simulink model "HANcoder_E407_TTA_Controller_v3"  (R2018b)
settings: Solver=FixedStepDiscrete  StartTime=0.0  StopTime=1  FixedStep=0.01  RelTol=1e-3
PreLoadFcn:
  | librarySetup
  | eval([bdroot,'_startup']) %Calling [modelName]_startup.m
values from neighbouring files (symbols this model uses):
  basic_cycle_duration_bc0 = TM_Reset_Board   + COMP_duration    (= 212)    [HANcoder_E407_TTA_Controller_v3_startup.m]
  basic_cycle_duration_bc1 = TM_Reset_Var_bc1 + COMP_duration    (= 288)    [HANcoder_E407_TTA_Controller_v3_startup.m]
  comm_delay_estimation1 = round(comm_delay_measured1*hardware_granularity/frequency_IRQ)    [HANcoder_E407_TTA_Controller_v3_startup.m]
  comm_delay_estimation2 = round(comm_delay_measured2*hardware_granularity/frequency_IRQ)    [HANcoder_E407_TTA_Controller_v3_startup.m]
  COMM_Period = 40    [HANcoder_E407_TTA_Controller_v3_startup.m]
  COMM_Phase1 = 5    [HANcoder_E407_TTA_Controller_v3_startup.m]
  COMM_Phase2 = 8    [HANcoder_E407_TTA_Controller_v3_startup.m]
  COMP_duration = 4    [HANcoder_E407_TTA_Controller_v3_startup.m]
  Controller1_Board = 1    [HANcoder_E407_TTA_Controller_v3_startup.m]
  Controller2_Board = 2    [HANcoder_E407_TTA_Controller_v3_startup.m]
  Controller3_Board = 3    [HANcoder_E407_TTA_Controller_v3_startup.m]
  delta_a_set = Simulink.Parameter    [HANcoder_E407_TTA_Controller_v3_startup.m]
  delta_f_set = Simulink.Parameter    [HANcoder_E407_TTA_Controller_v3_startup.m]
  delta_max = 1    [HANcoder_E407_TTA_Controller_v3_startup.m]
  delta_min = -1    [HANcoder_E407_TTA_Controller_v3_startup.m]
  delta_precision = 6    [HANcoder_E407_TTA_Controller_v3_startup.m]
  e_width = 0.1    [HANcoder_E407_TTA_Controller_v3_startup.m]
  frequency_IRQ = 100    [HANcoder_E407_TTA_Controller_v3_startup.m]
  HANtuneOverride = Simulink.Parameter    [HANcoder_E407_TTA_Controller_v3_startup.m]
  hardware_granularity = 1000000    [HANcoder_E407_TTA_Controller_v3_startup.m]
  I_a = 2.25    [HANcoder_E407_TTA_Controller_v3_startup.m]
  I_f = 2.25    [HANcoder_E407_TTA_Controller_v3_startup.m]
  idle_time_init = basic_cycle_duration_bc0 + basic_cycle_duration_bc1    (= 500)    [HANcoder_E407_TTA_Controller_v3_startup.m]
  Input_Gen_Board = 4    [HANcoder_E407_TTA_Controller_v3_startup.m]
  LA_Clock_Gr = 1    [HANcoder_E407_TTA_Controller_v3_startup.m]
  LA_COMM_Err = 0    [HANcoder_E407_TTA_Controller_v3_startup.m]
  LA_MEX_Flag = 0    [HANcoder_E407_TTA_Controller_v3_startup.m]
  LA_Task_Act = 1    [HANcoder_E407_TTA_Controller_v3_startup.m]
  m_v = 100.0    (= 100)    [HANcoder_E407_TTA_Controller_v3_startup.m]
  Master_Role = 1    [HANcoder_E407_TTA_Controller_v3_startup.m]
  matrix_cycle_duration = basic_cycle_duration_bc0 + basic_cycle_duration_bc1    (= 500)    [HANcoder_E407_TTA_Controller_v3_startup.m]
  matrix_rows = 2    [HANcoder_E407_TTA_Controller_v3_startup.m]
  max_num_msgs_CAN1 = 2^Tx_bit_number-1    (= 7)    [HANcoder_E407_TTA_Controller_v3_startup.m]
  max_num_msgs_CAN2 = max_num_msgs_CAN1    (= 7)    [HANcoder_E407_TTA_Controller_v3_startup.m]
  OutControl1_ID = 23    [HANcoder_E407_TTA_Controller_v3_startup.m]
  OutControl2_ID = 24    [HANcoder_E407_TTA_Controller_v3_startup.m]
  OutEmulator_ID = 25    [HANcoder_E407_TTA_Controller_v3_startup.m]
  R_al = 0.10    (= 0.1)    [HANcoder_E407_TTA_Controller_v3_startup.m]
  R_ar = 0.10    (= 0.1)    [HANcoder_E407_TTA_Controller_v3_startup.m]
  R_fl = 0.10    (= 0.1)    [HANcoder_E407_TTA_Controller_v3_startup.m]
  R_fr = 0.10    (= 0.1)    [HANcoder_E407_TTA_Controller_v3_startup.m]
  SensorValues_ID = 22    [HANcoder_E407_TTA_Controller_v3_startup.m]
  SetValues_ID = 21    [HANcoder_E407_TTA_Controller_v3_startup.m]
  Slave_Role = 2    [HANcoder_E407_TTA_Controller_v3_startup.m]
  speed_k_d = Simulink.Parameter    [HANcoder_E407_TTA_Controller_v3_startup.m]
  speed_k_i = Simulink.Parameter    [HANcoder_E407_TTA_Controller_v3_startup.m]
  speed_k_p = Simulink.Parameter    [HANcoder_E407_TTA_Controller_v3_startup.m]
  speed_max = 10    [HANcoder_E407_TTA_Controller_v3_startup.m]
  speed_min = -10    [HANcoder_E407_TTA_Controller_v3_startup.m]
  speed_precision = 3    [HANcoder_E407_TTA_Controller_v3_startup.m]
  Sync_ID = 1    [HANcoder_E407_TTA_Controller_v3_startup.m]
  tau_max = 5    [HANcoder_E407_TTA_Controller_v3_startup.m]
  tau_min = -5    [HANcoder_E407_TTA_Controller_v3_startup.m]
  tau_range = abs(tau_max) + abs(tau_min)    [HANcoder_E407_TTA_Controller_v3_startup.m]
  theta_max = 2    [HANcoder_E407_TTA_Controller_v3_startup.m]
  theta_min = -2    [HANcoder_E407_TTA_Controller_v3_startup.m]
  theta_precision = 5    [HANcoder_E407_TTA_Controller_v3_startup.m]
  Tl_a = 0.6    [HANcoder_E407_TTA_Controller_v3_startup.m]
  Tl_f = 0.6    [HANcoder_E407_TTA_Controller_v3_startup.m]
  TM_Check_Output_Control1 = TM_COMM_Output_Control1 + COMM_duration    (= 188)    [HANcoder_E407_TTA_Controller_v3_startup.m]
  TM_Check_Output_Control2 = TM_COMM_Output_Control2 + COMM_duration    (= 232)    [HANcoder_E407_TTA_Controller_v3_startup.m]
  TM_Check_Output_Emulator = TM_COMM_Output_Emulator + COMM_duration    (= 280)    [HANcoder_E407_TTA_Controller_v3_startup.m]
  TM_Check_Sensor_Values = TM_COMM_Sensor_Values + COMM_duration    (= 132)    [HANcoder_E407_TTA_Controller_v3_startup.m]
  TM_Check_Set_Values = TM_COMM_Set_Values + COMM_duration    (= 88)    [HANcoder_E407_TTA_Controller_v3_startup.m]
  TM_Check_Sync = TM_COMM_Sync   + COMM_duration    (= 40)    [HANcoder_E407_TTA_Controller_v3_startup.m]
  TM_Check_TOuts = TM_Count_Vote3 + COMP_duration    (= 196)    [HANcoder_E407_TTA_Controller_v3_startup.m]
  TM_Check_Vote1 = TM_COMM_Vote1  + COMM_duration    (= 92)    [HANcoder_E407_TTA_Controller_v3_startup.m]
  TM_Check_Vote2 = TM_COMM_Vote2  + COMM_duration    (= 140)    [HANcoder_E407_TTA_Controller_v3_startup.m]
  TM_Check_Vote3 = TM_COMM_Vote3  + COMM_duration    (= 188)    [HANcoder_E407_TTA_Controller_v3_startup.m]
  TM_COMM_Output_Control1 = TM_Velocity + COMP_duration    (= 148)    [HANcoder_E407_TTA_Controller_v3_startup.m]
  TM_COMM_Output_Control2 = TM_Check_Output_Control1 + COMP_duration    (= 192)    [HANcoder_E407_TTA_Controller_v3_startup.m]
  TM_COMM_Output_Emulator = TM_TMR + COMP_duration    (= 240)    [HANcoder_E407_TTA_Controller_v3_startup.m]
  TM_COMM_Sensor_Values = TM_Check_Set_Values + COMP_duration    (= 92)    [HANcoder_E407_TTA_Controller_v3_startup.m]
  TM_COMM_Set_Values = TM_Update_LT + COMP_duration    (= 48)    [HANcoder_E407_TTA_Controller_v3_startup.m]
  TM_COMM_Sync = basic_cycle_start    (= 0)    [HANcoder_E407_TTA_Controller_v3_startup.m]
  TM_COMM_Vote1 = TM_Vote_Dec    + COMP_duration    (= 52)    [HANcoder_E407_TTA_Controller_v3_startup.m]
  TM_COMM_Vote2 = TM_Count_Vote1 + COMP_duration    (= 100)    [HANcoder_E407_TTA_Controller_v3_startup.m]
  TM_COMM_Vote3 = TM_Count_Vote2 + COMP_duration    (= 148)    [HANcoder_E407_TTA_Controller_v3_startup.m]
  TM_Count_Vote1 = TM_Check_Vote1 + COMP_duration    (= 96)    [HANcoder_E407_TTA_Controller_v3_startup.m]
  TM_Count_Vote2 = TM_Check_Vote2 + COMP_duration    (= 144)    [HANcoder_E407_TTA_Controller_v3_startup.m]
  TM_Count_Vote3 = TM_Check_Vote3 + COMP_duration    (= 192)    [HANcoder_E407_TTA_Controller_v3_startup.m]
  TM_Data_bc0 = TM_COMM_Sync    (= 0)    [HANcoder_E407_TTA_Controller_v3_startup.m]
  TM_Data_bc1 = TM_Data_bc0(1:3)    [HANcoder_E407_TTA_Controller_v3_startup.m]
  TM_New_Master = TM_Check_TOuts + COMP_duration    (= 200)    [HANcoder_E407_TTA_Controller_v3_startup.m]
  TM_Reset_Board = TM_Reset_Var   + COMP_duration    (= 208)    [HANcoder_E407_TTA_Controller_v3_startup.m]
  TM_Reset_Var = TM_New_Master  + COMP_duration    (= 204)    [HANcoder_E407_TTA_Controller_v3_startup.m]
  TM_Reset_Var_bc1 = TM_Check_Output_Emulator + COMP_duration    (= 284)    [HANcoder_E407_TTA_Controller_v3_startup.m]
  TM_Steer = TM_Check_Sensor_Values + COMP_duration    (= 136)    [HANcoder_E407_TTA_Controller_v3_startup.m]
  TM_TMR = TM_Check_Output_Control2 + COMP_duration    (= 236)    [HANcoder_E407_TTA_Controller_v3_startup.m]
  TM_Torque = TM_Steer + COMP_duration    (= 140)    [HANcoder_E407_TTA_Controller_v3_startup.m]
  TM_Type_bc0 = COMM    (= 0)    [HANcoder_E407_TTA_Controller_v3_startup.m]
  TM_Type_bc1 = TM_Type_bc0(1:3)    [HANcoder_E407_TTA_Controller_v3_startup.m]
  TM_Update_LT = TM_Check_Sync  + COMP_duration    (= 44)    [HANcoder_E407_TTA_Controller_v3_startup.m]
  TM_Velocity = TM_Torque + COMP_duration    (= 144)    [HANcoder_E407_TTA_Controller_v3_startup.m]
  TM_Vote_Dec = TM_Update_LT   + COMP_duration    (= 48)    [HANcoder_E407_TTA_Controller_v3_startup.m]
  torque_a_k_d = Simulink.Parameter    [HANcoder_E407_TTA_Controller_v3_startup.m]
  torque_a_k_i = Simulink.Parameter    [HANcoder_E407_TTA_Controller_v3_startup.m]
  torque_a_k_p = Simulink.Parameter    [HANcoder_E407_TTA_Controller_v3_startup.m]
  torque_f_k_d = Simulink.Parameter    [HANcoder_E407_TTA_Controller_v3_startup.m]
  torque_f_k_i = Simulink.Parameter    [HANcoder_E407_TTA_Controller_v3_startup.m]
  torque_f_k_p = Simulink.Parameter    [HANcoder_E407_TTA_Controller_v3_startup.m]
  torque_precision = 4    [HANcoder_E407_TTA_Controller_v3_startup.m]
  v_set = Simulink.Parameter    [HANcoder_E407_TTA_Controller_v3_startup.m]
  Vehicle_Em_Board = 5    [HANcoder_E407_TTA_Controller_v3_startup.m]
  Vote1_ID = 11    [HANcoder_E407_TTA_Controller_v3_startup.m]
  Vote2_ID = 12    [HANcoder_E407_TTA_Controller_v3_startup.m]
  Vote3_ID = 13    [HANcoder_E407_TTA_Controller_v3_startup.m]
undefined symbols (not defined in the file or in its folder): A0, A1, A2, A3, A4, CON2
libraries: hdlsllib x352, HANcoder_STM32_Target x25, simulink x3, simulink_extras x1
(part 18 of 32)

== system HANcoder_E407_TTA_Controller_v3/HANcoder STM32 Target - E407-STM32 algorithm/Global Ticks Increment/CAN Management/Matrix Cycle Manager/Controller Matrix Cycle/controller basic cycle 0/COMP Task - Vote3 check/Process_Messages/Demux message CAN1 and check coherence1 ==
  CAN2_Rx_msg : Inport  OutDataTypeStr=Bus: msg_buffer_type
  expected_board_id : Inport  Port=2
  Enable : EnablePort
  Bus Creator : BusCreator  Inputs=8  OutDataTypeStr=Bus: msg_buffer_type
  Bus Selector : BusSelector  OutputSignals=Buffer_1,Buffer_2,Buffer_3,Buffer_4,Buffer_5,Buffer_6,Buffer_7,Buffer_8
  Cast To Double : DataTypeConversion  OutDataTypeStr=double
  Constant : Constant  Value=0  OutDataTypeStr=uint8
  Equal : RelationalOperator  Operator===  OutDataTypeStr=boolean  RndMeth=Simplest
  Subsystem : Subsystem
  Terminator : Terminator
  Terminator1 : Terminator
  msg_count>2_DEBUG : Subsystem
  CAN2_msg_coherent : Outport  OutputWhenDisabled=reset  InitialOutput=0
  Msg_Count_CAN2 : Outport  Port=2
  CAN2_msg : Outport  Port=3  OutDataTypeStr=Bus: msg_buffer_type
  wires:
  Bus Selector/2 -> Bus Creator/2  "<Buffer_2>"
  Bus Selector/3 -> Bus Creator/3  "<Buffer_3>"
  CAN2_Rx_msg/1 -> Bus Selector/1
  Equal/1 -> CAN2_msg_coherent/1
  expected_board_id/1 -> Equal/2
  Bus Selector/6 -> Bus Creator/6  "<Buffer_6>"
  Bus Selector/5 -> Bus Creator/5  "<Buffer_5>"
  Bus Selector/7 -> Bus Creator/7  "<Buffer_7>"
  Bus Selector/8 -> Bus Creator/8  "<Buffer_8>"
  Bus Selector/4 -> Bus Creator/4  "<Buffer_4>"
  Subsystem/3(board_id) -> Equal/1  "Rx_id_vote3_CAN2"
  Bus Selector/1 -> Cast To Double/1, Subsystem/1(Msg_Temporal_Data)  "<Buffer_1>"
  Subsystem/2(msg_count) -> Msg_Count_CAN2/1, msg_count>2_DEBUG/1(msg_c)  "Rx_mc_vote3_CAN2"
  Bus Creator/1 -> CAN2_msg/1
  Constant/1 -> Bus Creator/1
  Subsystem/1(basic_cycle) -> Terminator/1  "Rx_bc_vote3_CAN2"
  Cast To Double/1 -> Terminator1/1  "Rx_temporal_vote3_CAN2"

== system HANcoder_E407_TTA_Controller_v3/HANcoder STM32 Target - E407-STM32 algorithm/Global Ticks Increment/CAN Management/Matrix Cycle Manager/Controller Matrix Cycle/controller basic cycle 1/COMM Task - Output Control1/Reception substasks/RX buffers update ==
  note: CAN2
  note: CAN1
  note: Reception end - Set RxID and Reset CAN buffer flags
  note: Reset Rx buffers
  note: Wait until new message
      | arrives
  note: Reception ID
      |    Sync Msg: 1
      |    Vote Node 1: 11
      |    Vote Node 2: 12
      |    Vote Node 3: 13
  note: Reset RX Buffer Flag
  note: Wait until new message
      | arrives
  note: Reception ID
      |    Sync Msg: 1
      |    Vote Node 1: 11
      |    Vote Node 2: 12
      |    Vote Node 3: 13
  note: Reset RX Buffer Flag
  Rx_ID : Inport
  Enable : EnablePort
  Cast13 : DataTypeConversion  OutDataTypeStr=uint32
  Cast14 : DataTypeConversion  OutDataTypeStr=boolean
  Cast15 : DataTypeConversion  OutDataTypeStr=uint8
  Cast3 : DataTypeConversion  OutDataTypeStr=uint32
  Cast5 : DataTypeConversion  OutDataTypeStr=boolean
  Cast6 : DataTypeConversion  OutDataTypeStr=uint8
  Data Store Write : DataStoreWrite  DataStoreName=Msg_Rx
  Data Store Write11 : DataStoreWrite  DataStoreName=RxID_CAN2
  Data Store Write12 : DataStoreWrite  DataStoreName=Rx_State_CAN2
  Data Store Write2 : DataStoreWrite  DataStoreName=New_Msg_Ready_CAN1
  Data Store Write3 : DataStoreWrite  DataStoreName=new_msg_Rx
  Data Store Write6 : DataStoreWrite  DataStoreName=RxID_CAN1
  Data Store Write7 : DataStoreWrite  DataStoreName=Rx_State_CAN1
  Data Store Write9 : DataStoreWrite  DataStoreName=New_Msg_Ready_CAN2
  RESET1 : Constant  Value=0
  RESET2 : Constant  Value=0
  RESET_CAN1_new_buffer : Constant  Value=0
  RESET_CAN2_new_buffer : Constant  Value=0
  RESET_Msg_Rx : Constant  Value=0  OutDataTypeStr=Bus: msg_buffer_type
  RESET_new_msg_Rx : Constant  Value=0  OutDataTypeStr=boolean
  wires:
  Cast3/1 -> Data Store Write6/1
  RESET1/1 -> Cast5/1
  Cast5/1 -> Data Store Write2/1
  RESET_Msg_Rx/1 -> Data Store Write/1
  RESET_new_msg_Rx/1 -> Data Store Write3/1
  RESET_CAN1_new_buffer/1 -> Cast6/1
  Cast6/1 -> Data Store Write7/1
  Cast15/1 -> Data Store Write12/1
  RESET_CAN2_new_buffer/1 -> Cast15/1
  Cast14/1 -> Data Store Write9/1
  RESET2/1 -> Cast14/1
  Rx_ID/1 -> Cast13/1, Cast3/1
  Cast13/1 -> Data Store Write11/1

== system HANcoder_E407_TTA_Controller_v3/HANcoder STM32 Target - E407-STM32 algorithm/Global Ticks Increment/CAN Management/Matrix Cycle Manager/Controller Matrix Cycle/controller basic cycle 1/COMM Task - Output Control1/Transmission subtasks/Check msg transmission CAN1 ==
  note: In the next tick, a message will be
      | sent through CAN1
  note: A message should be sent during
      | this tick through CAN1
  note: The TX buffers are updated one tick
      | before the message is sent
  Local Time : Inport
  Time Mark : Inport  Port=2
  Tx_ID : Inport  Port=3
  Value Domain Msg : Inport  Port=4
  Enable : EnablePort
  Constant11 : Constant  Value=0
  Constant22 : Constant
  Constant24 : Constant  Value=COMM_Phase1
  Constant27 : Constant  Value=COMM_Phase1
  Constant8 : Constant  Value=0
  Equal4 : RelationalOperator  Operator===  OutDataTypeStr=boolean  RndMeth=Simplest
  Equal7 : RelationalOperator  Operator===  OutDataTypeStr=boolean  RndMeth=Simplest
  Minus : Sum  Inputs=++-
  Minus1 : Sum  Inputs=+-
  Mod : Math  Operator=mod  SaturateOnIntegerOverflow=on
  Mod1 : Math  Operator=mod  SaturateOnIntegerOverflow=on
  TX buffer update CAN1 : Subsystem  Priority=20
  Send CAN1 : Outport  OutputWhenDisabled=reset  InitialOutput=0
  wires:
  Constant8/1 -> Equal4/2
  Equal7/1 -> Send CAN1/1
  Constant11/1 -> Equal7/2
  Minus1/1 -> Mod1/1
  Mod/1 -> Equal4/1
  Constant24/1 -> Mod/2
  Value Domain Msg/1 -> TX buffer update CAN1/2(Msg_Value_Data)
  Minus/1 -> Mod/1
  Constant27/1 -> Mod1/2
  Mod1/1 -> Equal7/1
  Tx_ID/1 -> TX buffer update CAN1/1(Tx_ID)
  Local Time/1 -> Minus/1, Minus1/1
  Constant22/1 -> Minus/2
  Equal4/1 -> TX buffer update CAN1/Enable
  Time Mark/1 -> Minus/3, Minus1/2

== system HANcoder_E407_TTA_Controller_v3/HANcoder STM32 Target - E407-STM32 algorithm/Global Ticks Increment/CAN Management/Matrix Cycle Manager/Controller Matrix Cycle/controller basic cycle 1/COMM Task - Output Control1/Transmission subtasks/Check msg transmission CAN2 ==
  note: The TX buffers are updated one tick
      | before the message is sent
  note: A message should be sent during
      | this tick through CAN2
  note: In the next tick, a message will be
      | sent through CAN2
  Local Time : Inport
  Time Mark : Inport  Port=2
  Tx_ID : Inport  Port=3
  Value Domain Msg : Inport  Port=4
  Enable : EnablePort
  Constant11 : Constant  Value=0
  Constant22 : Constant
  Constant24 : Constant  Value=COMM_Phase2
  Constant27 : Constant  Value=COMM_Phase2
  Constant8 : Constant  Value=0
  Equal4 : RelationalOperator  Operator===  OutDataTypeStr=boolean  RndMeth=Simplest
  Equal7 : RelationalOperator  Operator===  OutDataTypeStr=boolean  RndMeth=Simplest
  Minus : Sum  Inputs=++-
  Minus1 : Sum  Inputs=+-
  Mod : Math  Operator=mod  SaturateOnIntegerOverflow=on
  Mod1 : Math  Operator=mod  SaturateOnIntegerOverflow=on
  TX buffer update CAN2 : Subsystem  Priority=20
  Send CAN2 : Outport  OutputWhenDisabled=reset  InitialOutput=0
  wires:
  Time Mark/1 -> Minus1/2, Minus/3
  Equal4/1 -> TX buffer update CAN2/Enable
  Constant22/1 -> Minus/2
  Local Time/1 -> Minus1/1, Minus/1
  Tx_ID/1 -> TX buffer update CAN2/1(Tx_ID)
  Mod1/1 -> Equal7/1
  Constant27/1 -> Mod1/2
  Minus/1 -> Mod/1
  Value Domain Msg/1 -> TX buffer update CAN2/2(Msg_Value_Data)
  Constant24/1 -> Mod/2
  Mod/1 -> Equal4/1
  Minus1/1 -> Mod1/1
  Constant11/1 -> Equal7/2
  Equal7/1 -> Send CAN2/1
  Constant8/1 -> Equal4/2

== system HANcoder_E407_TTA_Controller_v3/HANcoder STM32 Target - E407-STM32 algorithm/Global Ticks Increment/CAN Management/Matrix Cycle Manager/Controller Matrix Cycle/controller basic cycle 1/COMM Task - Output Control1/Transmission subtasks/Msg_Value_Data_Encoded7 ==
  note: Value domain message encoding
      | <Warning!> The first buffer (from the top) is not used in transmission!
  Enable : EnablePort
  Bus Creator : BusCreator  Inputs=8  OutDataTypeStr=Bus: msg_buffer_type
  Cast : DataTypeConversion  OutDataTypeStr=uint8
  Cast1 : DataTypeConversion  OutDataTypeStr=uint8
  Constant : Constant  Value=0  OutDataTypeStr=uint8
  Constant{1,7,10,13} (4 alike) : Constant  Value=torque_precision
  Constant{5,8,11,14} (4 alike) : Constant  Value=tau_max
  Constant{6,9,12,15} (4 alike) : Constant  Value=tau_min
  Data Store Read : DataStoreRead  DataStoreName=torque_fr_set
  Data Store Read1 : DataStoreRead  DataStoreName=torque_fl_set
  Data Store Read2 : DataStoreRead  DataStoreName=torque_ar_set
  Data Store Read3 : DataStoreRead  DataStoreName=torque_al_set
  Data Store Read4 : DataStoreRead  DataStoreName=Error_SensorValues_NotRX
  Data Store Read5 : DataStoreRead  DataStoreName=Error_SetValues_NotRX
  float2uint1 : Subsystem
  float2uint2 : Subsystem
  float2uint3 : Subsystem
  float2uint4 : Subsystem
  Value_domain_msg : Outport
  wires:
  Bus Creator/1 -> Value_domain_msg/1
  Data Store Read5/1 -> Cast/1
  Data Store Read4/1 -> Cast1/1
  Cast/1 -> Bus Creator/6
  Cast1/1 -> Bus Creator/7
  Constant/1 -> Bus Creator/1, Bus Creator/8
  float2uint2/1(coded) -> Bus Creator/2
  float2uint1/1(coded) -> Bus Creator/3
  float2uint3/1(coded) -> Bus Creator/4
  float2uint4/1(coded) -> Bus Creator/5
  Data Store Read/1 -> float2uint2/2(magnitude)
  Constant1/1 -> float2uint2/1(precision)
  Constant5/1 -> float2uint2/3(magnitude_max)
  Constant6/1 -> float2uint2/4(magnitude_min)
  Constant9/1 -> float2uint1/4(magnitude_min)
  Constant8/1 -> float2uint1/3(magnitude_max)
  Constant7/1 -> float2uint1/1(precision)
  Data Store Read1/1 -> float2uint1/2(magnitude)
  Constant10/1 -> float2uint3/1(precision)
  Data Store Read2/1 -> float2uint3/2(magnitude)
  Constant11/1 -> float2uint3/3(magnitude_max)
  Constant12/1 -> float2uint3/4(magnitude_min)
  Constant13/1 -> float2uint4/1(precision)
  Data Store Read3/1 -> float2uint4/2(magnitude)
  Constant14/1 -> float2uint4/3(magnitude_max)
  Constant15/1 -> float2uint4/4(magnitude_min)

== system HANcoder_E407_TTA_Controller_v3/HANcoder STM32 Target - E407-STM32 algorithm/Global Ticks Increment/CAN Management/Matrix Cycle Manager/Controller Matrix Cycle/controller basic cycle 1/COMM Task - Output Control2/Reception substasks/RX buffers update ==
  note: Reset RX Buffer Flag
  note: Reception ID
      |    Sync Msg: 1
      |    Vote Node 1: 11
      |    Vote Node 2: 12
      |    Vote Node 3: 13
  note: Wait until new message
      | arrives
  note: Reset RX Buffer Flag
  note: Reception ID
      |    Sync Msg: 1
      |    Vote Node 1: 11
      |    Vote Node 2: 12
      |    Vote Node 3: 13
  note: Wait until new message
      | arrives
  note: Reset Rx buffers
  note: Reception end - Set RxID and Reset CAN buffer flags
  note: CAN1
  note: CAN2
  Rx_ID : Inport
  Enable : EnablePort
  Cast13 : DataTypeConversion  OutDataTypeStr=uint32
  Cast14 : DataTypeConversion  OutDataTypeStr=boolean
  Cast15 : DataTypeConversion  OutDataTypeStr=uint8
  Cast3 : DataTypeConversion  OutDataTypeStr=uint32
  Cast5 : DataTypeConversion  OutDataTypeStr=boolean
  Cast6 : DataTypeConversion  OutDataTypeStr=uint8
  Data Store Write : DataStoreWrite  DataStoreName=Msg_Rx
  Data Store Write11 : DataStoreWrite  DataStoreName=RxID_CAN2
  Data Store Write12 : DataStoreWrite  DataStoreName=Rx_State_CAN2
  Data Store Write2 : DataStoreWrite  DataStoreName=New_Msg_Ready_CAN1
  Data Store Write3 : DataStoreWrite  DataStoreName=new_msg_Rx
  Data Store Write6 : DataStoreWrite  DataStoreName=RxID_CAN1
  Data Store Write7 : DataStoreWrite  DataStoreName=Rx_State_CAN1
  Data Store Write9 : DataStoreWrite  DataStoreName=New_Msg_Ready_CAN2
  RESET1 : Constant  Value=0
  RESET2 : Constant  Value=0
  RESET_CAN1_new_buffer : Constant  Value=0
  RESET_CAN2_new_buffer : Constant  Value=0
  RESET_Msg_Rx : Constant  Value=0  OutDataTypeStr=Bus: msg_buffer_type
  RESET_new_msg_Rx : Constant  Value=0  OutDataTypeStr=boolean
  wires:
  Cast13/1 -> Data Store Write11/1
  Rx_ID/1 -> Cast3/1, Cast13/1
  RESET2/1 -> Cast14/1
  Cast14/1 -> Data Store Write9/1
  RESET_CAN2_new_buffer/1 -> Cast15/1
  Cast15/1 -> Data Store Write12/1
  Cast6/1 -> Data Store Write7/1
  RESET_CAN1_new_buffer/1 -> Cast6/1
  RESET_new_msg_Rx/1 -> Data Store Write3/1
  RESET_Msg_Rx/1 -> Data Store Write/1
  Cast5/1 -> Data Store Write2/1
  RESET1/1 -> Cast5/1
  Cast3/1 -> Data Store Write6/1

== system HANcoder_E407_TTA_Controller_v3/HANcoder STM32 Target - E407-STM32 algorithm/Global Ticks Increment/CAN Management/Matrix Cycle Manager/Controller Matrix Cycle/controller basic cycle 1/COMM Task - Output Control2/Transmission subtasks/Check msg transmission CAN1 ==
  note: The TX buffers are updated one tick
      | before the message is sent
  note: A message should be sent during
      | this tick through CAN1
  note: In the next tick, a message will be
      | sent through CAN1
  Local Time : Inport
  Time Mark : Inport  Port=2
  Tx_ID : Inport  Port=3
  Value Domain Msg : Inport  Port=4
  Enable : EnablePort
  Constant11 : Constant  Value=0
  Constant22 : Constant
  Constant24 : Constant  Value=COMM_Phase1
  Constant27 : Constant  Value=COMM_Phase1
  Constant8 : Constant  Value=0
  Equal4 : RelationalOperator  Operator===  OutDataTypeStr=boolean  RndMeth=Simplest
  Equal7 : RelationalOperator  Operator===  OutDataTypeStr=boolean  RndMeth=Simplest
  Minus : Sum  Inputs=++-
  Minus1 : Sum  Inputs=+-
  Mod : Math  Operator=mod  SaturateOnIntegerOverflow=on
  Mod1 : Math  Operator=mod  SaturateOnIntegerOverflow=on
  TX buffer update CAN1 : Subsystem  Priority=20
  Send CAN1 : Outport  OutputWhenDisabled=reset  InitialOutput=0
  wires:
  Time Mark/1 -> Minus1/2, Minus/3
  Equal4/1 -> TX buffer update CAN1/Enable
  Constant22/1 -> Minus/2
  Local Time/1 -> Minus1/1, Minus/1
  Tx_ID/1 -> TX buffer update CAN1/1(Tx_ID)
  Mod1/1 -> Equal7/1
  Constant27/1 -> Mod1/2
  Minus/1 -> Mod/1
  Value Domain Msg/1 -> TX buffer update CAN1/2(Msg_Value_Data)
  Constant24/1 -> Mod/2
  Mod/1 -> Equal4/1
  Minus1/1 -> Mod1/1
  Constant11/1 -> Equal7/2
  Equal7/1 -> Send CAN1/1
  Constant8/1 -> Equal4/2

== system HANcoder_E407_TTA_Controller_v3/HANcoder STM32 Target - E407-STM32 algorithm/Global Ticks Increment/CAN Management/Matrix Cycle Manager/Controller Matrix Cycle/controller basic cycle 1/COMM Task - Output Control2/Transmission subtasks/Check msg transmission CAN2 ==
  note: In the next tick, a message will be
      | sent through CAN2
  note: A message should be sent during
      | this tick through CAN2
  note: The TX buffers are updated one tick
      | before the message is sent
  Local Time : Inport
  Time Mark : Inport  Port=2
  Tx_ID : Inport  Port=3
  Value Domain Msg : Inport  Port=4
  Enable : EnablePort
  Constant11 : Constant  Value=0
  Constant22 : Constant
  Constant24 : Constant  Value=COMM_Phase2
  Constant27 : Constant  Value=COMM_Phase2
  Constant8 : Constant  Value=0
  Equal4 : RelationalOperator  Operator===  OutDataTypeStr=boolean  RndMeth=Simplest
  Equal7 : RelationalOperator  Operator===  OutDataTypeStr=boolean  RndMeth=Simplest
  Minus : Sum  Inputs=++-
  Minus1 : Sum  Inputs=+-
  Mod : Math  Operator=mod  SaturateOnIntegerOverflow=on
  Mod1 : Math  Operator=mod  SaturateOnIntegerOverflow=on
  TX buffer update CAN2 : Subsystem  Priority=20
  Send CAN2 : Outport  OutputWhenDisabled=reset  InitialOutput=0
  wires:
  Constant8/1 -> Equal4/2
  Equal7/1 -> Send CAN2/1
  Constant11/1 -> Equal7/2
  Minus1/1 -> Mod1/1
  Mod/1 -> Equal4/1
  Constant24/1 -> Mod/2
  Value Domain Msg/1 -> TX buffer update CAN2/2(Msg_Value_Data)
  Minus/1 -> Mod/1
  Constant27/1 -> Mod1/2
  Mod1/1 -> Equal7/1
  Tx_ID/1 -> TX buffer update CAN2/1(Tx_ID)
  Local Time/1 -> Minus/1, Minus1/1
  Constant22/1 -> Minus/2
  Equal4/1 -> TX buffer update CAN2/Enable
  Time Mark/1 -> Minus/3, Minus1/2

== system HANcoder_E407_TTA_Controller_v3/HANcoder STM32 Target - E407-STM32 algorithm/Global Ticks Increment/CAN Management/Matrix Cycle Manager/Controller Matrix Cycle/controller basic cycle 1/COMM Task - Output Control2/Transmission subtasks/Msg_Value_Data_Encoded7 ==
  note: Value domain message encoding
      | <Warning!> The first buffer (from the top) is not used in transmission!
  Enable : EnablePort
  Bus Creator : BusCreator  Inputs=8  OutDataTypeStr=Bus: msg_buffer_type
  Cast : DataTypeConversion  OutDataTypeStr=uint8
  Cast1 : DataTypeConversion  OutDataTypeStr=uint8
  Constant : Constant  Value=0  OutDataTypeStr=uint8
  Constant{1,7,10,13} (4 alike) : Constant  Value=torque_precision
  Constant{5,8,11,14} (4 alike) : Constant  Value=tau_max
  Constant{6,9,12,15} (4 alike) : Constant  Value=tau_min
  Data Store Read : DataStoreRead  DataStoreName=torque_fr_set
  Data Store Read1 : DataStoreRead  DataStoreName=torque_fl_set
  Data Store Read2 : DataStoreRead  DataStoreName=torque_ar_set
  Data Store Read3 : DataStoreRead  DataStoreName=torque_al_set
  Data Store Read4 : DataStoreRead  DataStoreName=Error_SensorValues_NotRX
  Data Store Read5 : DataStoreRead  DataStoreName=Error_SetValues_NotRX
  float2uint1 : Subsystem
  float2uint2 : Subsystem
  float2uint3 : Subsystem
  float2uint4 : Subsystem
  Value_domain_msg : Outport
  wires:
  Constant15/1 -> float2uint4/4(magnitude_min)
  Constant14/1 -> float2uint4/3(magnitude_max)
  Data Store Read3/1 -> float2uint4/2(magnitude)
  Constant13/1 -> float2uint4/1(precision)
  Constant12/1 -> float2uint3/4(magnitude_min)
  Constant11/1 -> float2uint3/3(magnitude_max)
  Data Store Read2/1 -> float2uint3/2(magnitude)
  Constant10/1 -> float2uint3/1(precision)
  Data Store Read1/1 -> float2uint1/2(magnitude)
  Constant7/1 -> float2uint1/1(precision)
  Constant8/1 -> float2uint1/3(magnitude_max)
  Constant9/1 -> float2uint1/4(magnitude_min)
  Constant6/1 -> float2uint2/4(magnitude_min)
  Constant5/1 -> float2uint2/3(magnitude_max)
  Constant1/1 -> float2uint2/1(precision)
  Data Store Read/1 -> float2uint2/2(magnitude)
  float2uint4/1(coded) -> Bus Creator/5
  float2uint3/1(coded) -> Bus Creator/4
  float2uint1/1(coded) -> Bus Creator/3
  float2uint2/1(coded) -> Bus Creator/2
  Constant/1 -> Bus Creator/8, Bus Creator/1
  Cast1/1 -> Bus Creator/7
  Cast/1 -> Bus Creator/6
  Data Store Read4/1 -> Cast1/1
  Data Store Read5/1 -> Cast/1
  Bus Creator/1 -> Value_domain_msg/1

== system HANcoder_E407_TTA_Controller_v3/HANcoder STM32 Target - E407-STM32 algorithm/Global Ticks Increment/CAN Management/Matrix Cycle Manager/Controller Matrix Cycle/controller basic cycle 1/COMM Task - Output Emulator/Reception substasks/RX buffers update ==
  note: CAN2
  note: CAN1
  note: Reception end - Set RxID and Reset CAN buffer flags
  note: Reset Rx buffers
  note: Wait until new message
      | arrives
  note: Reception ID
      |    Sync Msg: 1
      |    Vote Node 1: 11
      |    Vote Node 2: 12
      |    Vote Node 3: 13
  note: Reset RX Buffer Flag
  note: Wait until new message
      | arrives
  note: Reception ID
      |    Sync Msg: 1
      |    Vote Node 1: 11
      |    Vote Node 2: 12
      |    Vote Node 3: 13
  note: Reset RX Buffer Flag
  Rx_ID : Inport
  Enable : EnablePort
  Cast13 : DataTypeConversion  OutDataTypeStr=uint32
  Cast14 : DataTypeConversion  OutDataTypeStr=boolean
  Cast15 : DataTypeConversion  OutDataTypeStr=uint8
  Cast3 : DataTypeConversion  OutDataTypeStr=uint32
  Cast5 : DataTypeConversion  OutDataTypeStr=boolean
  Cast6 : DataTypeConversion  OutDataTypeStr=uint8
  Data Store Write : DataStoreWrite  DataStoreName=Msg_Rx
  Data Store Write11 : DataStoreWrite  DataStoreName=RxID_CAN2
  Data Store Write12 : DataStoreWrite  DataStoreName=Rx_State_CAN2
  Data Store Write2 : DataStoreWrite  DataStoreName=New_Msg_Ready_CAN1
  Data Store Write3 : DataStoreWrite  DataStoreName=new_msg_Rx
  Data Store Write6 : DataStoreWrite  DataStoreName=RxID_CAN1
  Data Store Write7 : DataStoreWrite  DataStoreName=Rx_State_CAN1
  Data Store Write9 : DataStoreWrite  DataStoreName=New_Msg_Ready_CAN2
  RESET1 : Constant  Value=0
  RESET2 : Constant  Value=0
  RESET_CAN1_new_buffer : Constant  Value=0
  RESET_CAN2_new_buffer : Constant  Value=0
  RESET_Msg_Rx : Constant  Value=0  OutDataTypeStr=Bus: msg_buffer_type
  RESET_new_msg_Rx : Constant  Value=0  OutDataTypeStr=boolean
  wires:
  Cast3/1 -> Data Store Write6/1
  RESET1/1 -> Cast5/1
  Cast5/1 -> Data Store Write2/1
  RESET_Msg_Rx/1 -> Data Store Write/1
  RESET_new_msg_Rx/1 -> Data Store Write3/1
  RESET_CAN1_new_buffer/1 -> Cast6/1
  Cast6/1 -> Data Store Write7/1
  Cast15/1 -> Data Store Write12/1
  RESET_CAN2_new_buffer/1 -> Cast15/1
  Cast14/1 -> Data Store Write9/1
  RESET2/1 -> Cast14/1
  Rx_ID/1 -> Cast13/1, Cast3/1
  Cast13/1 -> Data Store Write11/1

== system HANcoder_E407_TTA_Controller_v3/HANcoder STM32 Target - E407-STM32 algorithm/Global Ticks Increment/CAN Management/Matrix Cycle Manager/Controller Matrix Cycle/controller basic cycle 1/COMM Task - Output Emulator/Transmission subtasks/Check msg transmission CAN1 ==
  note: In the next tick, a message will be
      | sent through CAN1
  note: A message should be sent during
      | this tick through CAN1
  note: The TX buffers are updated one tick
      | before the message is sent
  Local Time : Inport
  Time Mark : Inport  Port=2
  Tx_ID : Inport  Port=3
  Value Domain Msg : Inport  Port=4
  Enable : EnablePort
  Constant11 : Constant  Value=0
  Constant22 : Constant
  Constant24 : Constant  Value=COMM_Phase1
  Constant27 : Constant  Value=COMM_Phase1
  Constant8 : Constant  Value=0
  Equal4 : RelationalOperator  Operator===  OutDataTypeStr=boolean  RndMeth=Simplest
  Equal7 : RelationalOperator  Operator===  OutDataTypeStr=boolean  RndMeth=Simplest
  Minus : Sum  Inputs=++-
  Minus1 : Sum  Inputs=+-
  Mod : Math  Operator=mod  SaturateOnIntegerOverflow=on
  Mod1 : Math  Operator=mod  SaturateOnIntegerOverflow=on
  TX buffer update CAN1 : Subsystem  Priority=20
  Send CAN1 : Outport  OutputWhenDisabled=reset  InitialOutput=0
  wires:
  Constant8/1 -> Equal4/2
  Equal7/1 -> Send CAN1/1
  Constant11/1 -> Equal7/2
  Minus1/1 -> Mod1/1
  Mod/1 -> Equal4/1
  Constant24/1 -> Mod/2
  Value Domain Msg/1 -> TX buffer update CAN1/2(Msg_Value_Data)
  Minus/1 -> Mod/1
  Constant27/1 -> Mod1/2
  Mod1/1 -> Equal7/1
  Tx_ID/1 -> TX buffer update CAN1/1(Tx_ID)
  Local Time/1 -> Minus/1, Minus1/1
  Constant22/1 -> Minus/2
  Equal4/1 -> TX buffer update CAN1/Enable
  Time Mark/1 -> Minus/3, Minus1/2

== system HANcoder_E407_TTA_Controller_v3/HANcoder STM32 Target - E407-STM32 algorithm/Global Ticks Increment/CAN Management/Matrix Cycle Manager/Controller Matrix Cycle/controller basic cycle 1/COMM Task - Output Emulator/Transmission subtasks/Check msg transmission CAN2 ==
  note: The TX buffers are updated one tick
      | before the message is sent
  note: A message should be sent during
      | this tick through CAN2
  note: In the next tick, a message will be
      | sent through CAN2
  Local Time : Inport
  Time Mark : Inport  Port=2
  Tx_ID : Inport  Port=3
  Value Domain Msg : Inport  Port=4
  Enable : EnablePort
  Constant11 : Constant  Value=0
  Constant22 : Constant
  Constant24 : Constant  Value=COMM_Phase2
  Constant27 : Constant  Value=COMM_Phase2
  Constant8 : Constant  Value=0
  Equal4 : RelationalOperator  Operator===  OutDataTypeStr=boolean  RndMeth=Simplest
  Equal7 : RelationalOperator  Operator===  OutDataTypeStr=boolean  RndMeth=Simplest
  Minus : Sum  Inputs=++-
  Minus1 : Sum  Inputs=+-
  Mod : Math  Operator=mod  SaturateOnIntegerOverflow=on
  Mod1 : Math  Operator=mod  SaturateOnIntegerOverflow=on
  TX buffer update CAN2 : Subsystem  Priority=20
  Send CAN2 : Outport  OutputWhenDisabled=reset  InitialOutput=0
  wires:
  Time Mark/1 -> Minus1/2, Minus/3
  Equal4/1 -> TX buffer update CAN2/Enable
  Constant22/1 -> Minus/2
  Local Time/1 -> Minus1/1, Minus/1
  Tx_ID/1 -> TX buffer update CAN2/1(Tx_ID)
  Mod1/1 -> Equal7/1
  Constant27/1 -> Mod1/2
  Minus/1 -> Mod/1
  Value Domain Msg/1 -> TX buffer update CAN2/2(Msg_Value_Data)
  Constant24/1 -> Mod/2
  Mod/1 -> Equal4/1
  Minus1/1 -> Mod1/1
  Constant11/1 -> Equal7/2
  Equal7/1 -> Send CAN2/1
  Constant8/1 -> Equal4/2

== system HANcoder_E407_TTA_Controller_v3/HANcoder STM32 Target - E407-STM32 algorithm/Global Ticks Increment/CAN Management/Matrix Cycle Manager/Controller Matrix Cycle/controller basic cycle 1/COMM Task - Output Emulator/Transmission subtasks/Msg_Value_Data_Encoded ==
  note: Value domain message encoding
      | <Warning!> The first buffer (from the top) is not used in transmission!
  Enable : EnablePort
  Bus Creator : BusCreator  Inputs=8  OutDataTypeStr=Bus: msg_buffer_type
  Constant : Constant  Value=0  OutDataTypeStr=uint8
  Constant{7,10..11,14} (4 alike) : Constant  Value=tau_min
  Constant{5,8,12,15} (4 alike) : Constant  Value=torque_precision
  Constant{6,9,13,16} (4 alike) : Constant  Value=tau_max
  Data Store Read1 : DataStoreRead  DataStoreName=torque_fl_set
  Data Store Read2 : DataStoreRead  DataStoreName=torque_ar_set
  Data Store Read3 : DataStoreRead  DataStoreName=torque_al_set
  Data Store Read4 : DataStoreRead  DataStoreName=error_log_1
  Data Store Read5 : DataStoreRead  DataStoreName=error_log_2
  Data Store Read6 : DataStoreRead  DataStoreName=error_log_3
  Data Store Read7 : DataStoreRead  DataStoreName=torque_fr_set
  float2uint1 : Subsystem
  float2uint2 : Subsystem
  float2uint3 : Subsystem
  float2uint4 : Subsystem
  Value_domain_msg : Outport
  wires:
  Bus Creator/1 -> Value_domain_msg/1
  Data Store Read5/1 -> Bus Creator/7
  Data Store Read6/1 -> Bus Creator/8
  Constant/1 -> Bus Creator/1
  Data Store Read4/1 -> Bus Creator/6
  Data Store Read7/1 -> float2uint2/2(magnitude)
  Constant6/1 -> float2uint2/3(magnitude_max)
  Constant5/1 -> float2uint2/1(precision)
  Constant7/1 -> float2uint2/4(magnitude_min)
  float2uint2/1(coded) -> Bus Creator/2
  Constant10/1 -> float2uint1/4(magnitude_min)
  Constant8/1 -> float2uint1/1(precision)
  Constant9/1 -> float2uint1/3(magnitude_max)
  Data Store Read1/1 -> float2uint1/2(magnitude)
  Data Store Read2/1 -> float2uint3/2(magnitude)
  Constant13/1 -> float2uint3/3(magnitude_max)
  Constant12/1 -> float2uint3/1(precision)
  Constant11/1 -> float2uint3/4(magnitude_min)
  float2uint3/1(coded) -> Bus Creator/4
  Constant14/1 -> float2uint4/4(magnitude_min)
  Constant15/1 -> float2uint4/1(precision)
  Constant16/1 -> float2uint4/3(magnitude_max)
  Data Store Read3/1 -> float2uint4/2(magnitude)
  float2uint4/1(coded) -> Bus Creator/5
  float2uint1/1(coded) -> Bus Creator/3

== system HANcoder_E407_TTA_Controller_v3/HANcoder STM32 Target - E407-STM32 algorithm/Global Ticks Increment/CAN Management/Matrix Cycle Manager/Controller Matrix Cycle/controller basic cycle 1/COMM Task - Sensor_Values/Reception substasks/RX buffers update ==
  note: Reset RX Buffer Flag
  note: Reception ID
      |    Sync Msg: 1
      |    Vote Node 1: 11
      |    Vote Node 2: 12
      |    Vote Node 3: 13
  note: Wait until new message
      | arrives
  note: Reset RX Buffer Flag
  note: Reception ID
      |    Sync Msg: 1
      |    Vote Node 1: 11
      |    Vote Node 2: 12
      |    Vote Node 3: 13
  note: Wait until new message
      | arrives
  note: Reset Rx buffers
  note: Reception end - Set RxID and Reset CAN buffer flags
  note: CAN1
  note: CAN2
  Rx_ID : Inport
  Enable : EnablePort
  Cast13 : DataTypeConversion  OutDataTypeStr=uint32
  Cast14 : DataTypeConversion  OutDataTypeStr=boolean
  Cast15 : DataTypeConversion  OutDataTypeStr=uint8
  Cast3 : DataTypeConversion  OutDataTypeStr=uint32
  Cast5 : DataTypeConversion  OutDataTypeStr=boolean
  Cast6 : DataTypeConversion  OutDataTypeStr=uint8
  Data Store Write : DataStoreWrite  DataStoreName=Msg_Rx
  Data Store Write11 : DataStoreWrite  DataStoreName=RxID_CAN2
  Data Store Write12 : DataStoreWrite  DataStoreName=Rx_State_CAN2
  Data Store Write2 : DataStoreWrite  DataStoreName=New_Msg_Ready_CAN1
  Data Store Write3 : DataStoreWrite  DataStoreName=new_msg_Rx
  Data Store Write6 : DataStoreWrite  DataStoreName=RxID_CAN1
  Data Store Write7 : DataStoreWrite  DataStoreName=Rx_State_CAN1
  Data Store Write9 : DataStoreWrite  DataStoreName=New_Msg_Ready_CAN2
  RESET1 : Constant  Value=0
  RESET2 : Constant  Value=0
  RESET_CAN1_new_buffer : Constant  Value=0
  RESET_CAN2_new_buffer : Constant  Value=0
  RESET_Msg_Rx : Constant  Value=0  OutDataTypeStr=Bus: msg_buffer_type
  RESET_new_msg_Rx : Constant  Value=0  OutDataTypeStr=boolean
  wires:
  Cast13/1 -> Data Store Write11/1
  Rx_ID/1 -> Cast3/1, Cast13/1
  RESET2/1 -> Cast14/1
  Cast14/1 -> Data Store Write9/1
  RESET_CAN2_new_buffer/1 -> Cast15/1
  Cast15/1 -> Data Store Write12/1
  Cast6/1 -> Data Store Write7/1
  RESET_CAN1_new_buffer/1 -> Cast6/1
  RESET_new_msg_Rx/1 -> Data Store Write3/1
  RESET_Msg_Rx/1 -> Data Store Write/1
  Cast5/1 -> Data Store Write2/1
  RESET1/1 -> Cast5/1
  Cast3/1 -> Data Store Write6/1

== system HANcoder_E407_TTA_Controller_v3/HANcoder STM32 Target - E407-STM32 algorithm/Global Ticks Increment/CAN Management/Matrix Cycle Manager/Controller Matrix Cycle/controller basic cycle 1/COMM Task - Sensor_Values/Transmission subtasks/Check msg transmission CAN1 ==
  note: The TX buffers are updated one tick
      | before the message is sent
  note: A message should be sent during
      | this tick through CAN1
  note: In the next tick, a message will be
      | sent through CAN1
  Local Time : Inport
  Time Mark : Inport  Port=2
  Tx_ID : Inport  Port=3
  Value Domain Msg : Inport  Port=4
  Enable : EnablePort
  Constant11 : Constant  Value=0
  Constant22 : Constant
  Constant24 : Constant  Value=COMM_Phase1
  Constant27 : Constant  Value=COMM_Phase1
  Constant8 : Constant  Value=0
  Equal4 : RelationalOperator  Operator===  OutDataTypeStr=boolean  RndMeth=Simplest
  Equal7 : RelationalOperator  Operator===  OutDataTypeStr=boolean  RndMeth=Simplest
  Minus : Sum  Inputs=++-
  Minus1 : Sum  Inputs=+-
  Mod : Math  Operator=mod  SaturateOnIntegerOverflow=on
  Mod1 : Math  Operator=mod  SaturateOnIntegerOverflow=on
  TX buffer update CAN1 : Subsystem  Priority=20
  Send CAN1 : Outport  OutputWhenDisabled=reset  InitialOutput=0
  wires:
  Time Mark/1 -> Minus1/2, Minus/3
  Equal4/1 -> TX buffer update CAN1/Enable
  Constant22/1 -> Minus/2
  Local Time/1 -> Minus1/1, Minus/1
  Tx_ID/1 -> TX buffer update CAN1/1(Tx_ID)
  Mod1/1 -> Equal7/1
  Constant27/1 -> Mod1/2
  Minus/1 -> Mod/1
  Value Domain Msg/1 -> TX buffer update CAN1/2(Msg_Value_Data)
  Constant24/1 -> Mod/2
  Mod/1 -> Equal4/1
  Minus1/1 -> Mod1/1
  Constant11/1 -> Equal7/2
  Equal7/1 -> Send CAN1/1
  Constant8/1 -> Equal4/2

== system HANcoder_E407_TTA_Controller_v3/HANcoder STM32 Target - E407-STM32 algorithm/Global Ticks Increment/CAN Management/Matrix Cycle Manager/Controller Matrix Cycle/controller basic cycle 1/COMM Task - Sensor_Values/Transmission subtasks/Check msg transmission CAN2 ==
  note: In the next tick, a message will be
      | sent through CAN2
  note: A message should be sent during
      | this tick through CAN2
  note: The TX buffers are updated one tick
      | before the message is sent
  Local Time : Inport
  Time Mark : Inport  Port=2
  Tx_ID : Inport  Port=3
  Value Domain Msg : Inport  Port=4
  Enable : EnablePort
  Constant11 : Constant  Value=0
  Constant22 : Constant
  Constant24 : Constant  Value=COMM_Phase2
  Constant27 : Constant  Value=COMM_Phase2
  Constant8 : Constant  Value=0
  Equal4 : RelationalOperator  Operator===  OutDataTypeStr=boolean  RndMeth=Simplest
  Equal7 : RelationalOperator  Operator===  OutDataTypeStr=boolean  RndMeth=Simplest
  Minus : Sum  Inputs=++-
  Minus1 : Sum  Inputs=+-
  Mod : Math  Operator=mod  SaturateOnIntegerOverflow=on
  Mod1 : Math  Operator=mod  SaturateOnIntegerOverflow=on
  TX buffer update CAN2 : Subsystem  Priority=20
  Send CAN2 : Outport  OutputWhenDisabled=reset  InitialOutput=0
  wires:
  Constant8/1 -> Equal4/2
  Equal7/1 -> Send CAN2/1
  Constant11/1 -> Equal7/2
  Minus1/1 -> Mod1/1
  Mod/1 -> Equal4/1
  Constant24/1 -> Mod/2
  Value Domain Msg/1 -> TX buffer update CAN2/2(Msg_Value_Data)
  Minus/1 -> Mod/1
  Constant27/1 -> Mod1/2
  Mod1/1 -> Equal7/1
  Tx_ID/1 -> TX buffer update CAN2/1(Tx_ID)
  Local Time/1 -> Minus/1, Minus1/1
  Constant22/1 -> Minus/2
  Equal4/1 -> TX buffer update CAN2/Enable
  Time Mark/1 -> Minus/3, Minus1/2

== system HANcoder_E407_TTA_Controller_v3/HANcoder STM32 Target - E407-STM32 algorithm/Global Ticks Increment/CAN Management/Matrix Cycle Manager/Controller Matrix Cycle/controller basic cycle 1/COMM Task - Sensor_Values/Transmission subtasks/Msg_Value_Data_Encoded6 ==
  note: <!> This is properly defined in vehicle emulator matrix cycle
  note: Value domain message encoding
      | <Warning!> The first buffer (from the top) is not used in transmission!
  Enable : EnablePort
  Bus Creator : BusCreator  Inputs=8  OutDataTypeStr=Bus: msg_buffer_type
  Constant : Constant  Value=0  OutDataTypeStr=uint8
  Constant{1,7,10,13} (4 alike) : Constant  Value=theta_precision
  Constant{5,8,11,14} (4 alike) : Constant  Value=theta_max
  Constant{6,9,12,15} (4 alike) : Constant  Value=theta_min
  Constant{2..4,16} (4 alike) : Constant  Value=0
  float2uint1 : Subsystem
  float2uint2 : Subsystem
  float2uint3 : Subsystem
  float2uint4 : Subsystem
  Value_domain_msg : Outport
  wires:
  Bus Creator/1 -> Value_domain_msg/1
  Constant2/1 -> float2uint2/2(magnitude)
  Constant1/1 -> float2uint2/1(precision)
  Constant/1 -> Bus Creator/1, Bus Creator/6, Bus Creator/7, Bus Creator/8
  float2uint2/1(coded) -> Bus Creator/2
  Constant5/1 -> float2uint2/3(magnitude_max)
  Constant6/1 -> float2uint2/4(magnitude_min)
  Constant9/1 -> float2uint1/4(magnitude_min)
  Constant8/1 -> float2uint1/3(magnitude_max)
  Constant7/1 -> float2uint1/1(precision)
  Constant3/1 -> float2uint1/2(magnitude)
  float2uint1/1(coded) -> Bus Creator/3
  Constant4/1 -> float2uint3/2(magnitude)
  Constant10/1 -> float2uint3/1(precision)
  Constant11/1 -> float2uint3/3(magnitude_max)
  Constant12/1 -> float2uint3/4(magnitude_min)
  float2uint3/1(coded) -> Bus Creator/4
  Constant15/1 -> float2uint4/4(magnitude_min)
  Constant14/1 -> float2uint4/3(magnitude_max)
  Constant13/1 -> float2uint4/1(precision)
  Constant16/1 -> float2uint4/2(magnitude)
  float2uint4/1(coded) -> Bus Creator/5

== system HANcoder_E407_TTA_Controller_v3/HANcoder STM32 Target - E407-STM32 algorithm/Global Ticks Increment/CAN Management/Matrix Cycle Manager/Controller Matrix Cycle/controller basic cycle 1/COMM Task - Set_Values/Reception substasks/RX buffers update ==
  note: CAN2
  note: CAN1
  note: Reception end - Set RxID and Reset CAN buffer flags
  note: Reset Rx buffers
  note: Wait until new message
      | arrives
  note: Reception ID
      |    Sync Msg: 1
      |    Vote Node 1: 11
      |    Vote Node 2: 12
      |    Vote Node 3: 13
  note: Reset RX Buffer Flag
  note: Wait until new message
      | arrives
  note: Reception ID
      |    Sync Msg: 1
      |    Vote Node 1: 11
      |    Vote Node 2: 12
      |    Vote Node 3: 13
  note: Reset RX Buffer Flag
  Rx_ID : Inport
  Enable : EnablePort
  Cast13 : DataTypeConversion  OutDataTypeStr=uint32
  Cast14 : DataTypeConversion  OutDataTypeStr=boolean
  Cast15 : DataTypeConversion  OutDataTypeStr=uint8
  Cast3 : DataTypeConversion  OutDataTypeStr=uint32
  Cast5 : DataTypeConversion  OutDataTypeStr=boolean
  Cast6 : DataTypeConversion  OutDataTypeStr=uint8
  Data Store Write : DataStoreWrite  DataStoreName=Msg_Rx
  Data Store Write11 : DataStoreWrite  DataStoreName=RxID_CAN2
  Data Store Write12 : DataStoreWrite  DataStoreName=Rx_State_CAN2
  Data Store Write2 : DataStoreWrite  DataStoreName=New_Msg_Ready_CAN1
  Data Store Write3 : DataStoreWrite  DataStoreName=new_msg_Rx
  Data Store Write6 : DataStoreWrite  DataStoreName=RxID_CAN1
  Data Store Write7 : DataStoreWrite  DataStoreName=Rx_State_CAN1
  Data Store Write9 : DataStoreWrite  DataStoreName=New_Msg_Ready_CAN2
  RESET1 : Constant  Value=0
  RESET2 : Constant  Value=0
  RESET_CAN1_new_buffer : Constant  Value=0
  RESET_CAN2_new_buffer : Constant  Value=0
  RESET_Msg_Rx : Constant  Value=0  OutDataTypeStr=Bus: msg_buffer_type
  RESET_new_msg_Rx : Constant  Value=0  OutDataTypeStr=boolean
  wires:
  Cast3/1 -> Data Store Write6/1
  RESET1/1 -> Cast5/1
  Cast5/1 -> Data Store Write2/1
  RESET_Msg_Rx/1 -> Data Store Write/1
  RESET_new_msg_Rx/1 -> Data Store Write3/1
  RESET_CAN1_new_buffer/1 -> Cast6/1
  Cast6/1 -> Data Store Write7/1
  Cast15/1 -> Data Store Write12/1
  RESET_CAN2_new_buffer/1 -> Cast15/1
  Cast14/1 -> Data Store Write9/1
  RESET2/1 -> Cast14/1
  Rx_ID/1 -> Cast13/1, Cast3/1
  Cast13/1 -> Data Store Write11/1

== system HANcoder_E407_TTA_Controller_v3/HANcoder STM32 Target - E407-STM32 algorithm/Global Ticks Increment/CAN Management/Matrix Cycle Manager/Controller Matrix Cycle/controller basic cycle 1/COMM Task - Set_Values/Transmission subtasks/Check msg transmission CAN1 ==
  note: In the next tick, a message will be
      | sent through CAN1
  note: A message should be sent during
      | this tick through CAN1
  note: The TX buffers are updated one tick
      | before the message is sent
  Local Time : Inport
  Time Mark : Inport  Port=2
  Tx_ID : Inport  Port=3
  Value Domain Msg : Inport  Port=4
  Enable : EnablePort
  Constant11 : Constant  Value=0
  Constant22 : Constant
  Constant24 : Constant  Value=COMM_Phase1
  Constant27 : Constant  Value=COMM_Phase1
  Constant8 : Constant  Value=0
  Equal4 : RelationalOperator  Operator===  OutDataTypeStr=boolean  RndMeth=Simplest
  Equal7 : RelationalOperator  Operator===  OutDataTypeStr=boolean  RndMeth=Simplest
  Minus : Sum  Inputs=++-
  Minus1 : Sum  Inputs=+-
  Mod : Math  Operator=mod  SaturateOnIntegerOverflow=on
  Mod1 : Math  Operator=mod  SaturateOnIntegerOverflow=on
  TX buffer update CAN1 : Subsystem  Priority=20
  Send CAN1 : Outport  OutputWhenDisabled=reset  InitialOutput=0
  wires:
  Constant8/1 -> Equal4/2
  Equal7/1 -> Send CAN1/1
  Constant11/1 -> Equal7/2
  Minus1/1 -> Mod1/1
  Mod/1 -> Equal4/1
  Constant24/1 -> Mod/2
  Value Domain Msg/1 -> TX buffer update CAN1/2(Msg_Value_Data)
  Minus/1 -> Mod/1
  Constant27/1 -> Mod1/2
  Mod1/1 -> Equal7/1
  Tx_ID/1 -> TX buffer update CAN1/1(Tx_ID)
  Local Time/1 -> Minus/1, Minus1/1
  Constant22/1 -> Minus/2
  Equal4/1 -> TX buffer update CAN1/Enable
  Time Mark/1 -> Minus/3, Minus1/2

== system HANcoder_E407_TTA_Controller_v3/HANcoder STM32 Target - E407-STM32 algorithm/Global Ticks Increment/CAN Management/Matrix Cycle Manager/Controller Matrix Cycle/controller basic cycle 1/COMM Task - Set_Values/Transmission subtasks/Check msg transmission CAN2 ==
  note: The TX buffers are updated one tick
      | before the message is sent
  note: A message should be sent during
      | this tick through CAN2
  note: In the next tick, a message will be
      | sent through CAN2
  Local Time : Inport
  Time Mark : Inport  Port=2
  Tx_ID : Inport  Port=3
  Value Domain Msg : Inport  Port=4
  Enable : EnablePort
  Constant11 : Constant  Value=0
  Constant22 : Constant
  Constant24 : Constant  Value=COMM_Phase2
  Constant27 : Constant  Value=COMM_Phase2
  Constant8 : Constant  Value=0
  Equal4 : RelationalOperator  Operator===  OutDataTypeStr=boolean  RndMeth=Simplest
  Equal7 : RelationalOperator  Operator===  OutDataTypeStr=boolean  RndMeth=Simplest
  Minus : Sum  Inputs=++-
  Minus1 : Sum  Inputs=+-
  Mod : Math  Operator=mod  SaturateOnIntegerOverflow=on
  Mod1 : Math  Operator=mod  SaturateOnIntegerOverflow=on
  TX buffer update CAN2 : Subsystem  Priority=20
  Send CAN2 : Outport  OutputWhenDisabled=reset  InitialOutput=0
  wires:
  Time Mark/1 -> Minus1/2, Minus/3
  Equal4/1 -> TX buffer update CAN2/Enable
  Constant22/1 -> Minus/2
  Local Time/1 -> Minus1/1, Minus/1
  Tx_ID/1 -> TX buffer update CAN2/1(Tx_ID)
  Mod1/1 -> Equal7/1
  Constant27/1 -> Mod1/2
  Minus/1 -> Mod/1
  Value Domain Msg/1 -> TX buffer update CAN2/2(Msg_Value_Data)
  Constant24/1 -> Mod/2
  Mod/1 -> Equal4/1
  Minus1/1 -> Mod1/1
  Constant11/1 -> Equal7/2
  Equal7/1 -> Send CAN2/1
  Constant8/1 -> Equal4/2
